simulink model "flightControlSystem"  (R2024b)
settings: Solver=ode3  StartTime=0  StopTime=TFinal  FixedStep=Ts  RelTol=1e-3  EnableMultiTasking=on
undefined symbols (not defined in the file): codertarget, completed, Controller, controller_selector, DiscIntNeverNeededParam, Discrete, distance, Estimator, filter_coef, g, gray, init, orient_ref, pos_ref, Sensors, Time, time_outside_line, Ts, var_acc_angle_N, var_bias_gyr_N, var_gyro_p_N, Vehicle, y
libraries: simulink x42, matrix_library x5, slpidlib x4, ctrlSharedLib x4, sharedtransform x3, parrotlib x1, visiongeotforms x1, simulink_extras x1
(part 3 of 3)

== system flightControlSystem/Control System/State Estimator/XY Position Estimator/EstimatorVelocity/AccelerationHandling ==
  dxy_estimin : Inport
  sensorIMU_datin : Inport  Port=2
  orient_estimin : Inport  Port=3
  Z_estimin : Inport  Port=4
  Add : Sum  Inputs=-+
  Bus Selector1 : BusSelector  OutputSignals=ddx,ddy,ddz
  Deactivate Acceleration If OF is not used due to low altitude : simulink/Logic and Bit Operations/Compare To Constant  relop=<=  const=Estimator.pos.opticalFlowZMax  OutDataTypeStr=boolean
  Logical Operator : Logic  Operator=OR  AllPortsSameDT=off  OutDataTypeStr=boolean
  Mux6 : Mux  Inputs=3
  Product : Product  Inputs=3
  Product1 : Product  Multiplication=Matrix(*)
  Rotation Angles to Direction Cosine Matrix : sharedtransform/Rotation Angles to Direction Cosine Matrix  rotationOrder=ZYX  aMode=aMode
  SelectPlanarddxy : Selector  InputPortWidth=3  IndexOptions=Index vector (dialog)  Indices=[1 2]  OutputSizes=1
  Selector : Selector  InputPortWidth=2  IndexOptions=Index vector (dialog)  Indices=1  OutputSizes=1
  Selector1 : Selector  InputPortWidth=2  IndexOptions=Index vector (dialog)  Indices=2  OutputSizes=1
  do not use acc if optical flow never available (Note OF@60Hz but ZOH to 200!) : simulink/Logic and Bit Operations/Compare To Constant  relop=~=  const=0  OutDataTypeStr=boolean
  do not use acc if optical flow never available (Note OF@60Hz but ZOH to 200!)1 : simulink/Logic and Bit Operations/Compare To Constant  relop=~=  const=0  OutDataTypeStr=boolean
  gainaccinput1 : Gain  OutDataTypeStr=single
  gravity : Constant  Value=[0 0 -g]
  acceleration_world : Outport  OutDataTypeStr=single  VectorParamsAs1DForOutWhenUnconnected=off
  wires:
  do not use acc if optical flow never available (Note OF@60Hz but ZOH to 200!)1/1 -> Logical Operator/2
  do not use acc if optical flow never available (Note OF@60Hz but ZOH to 200!)/1 -> Logical Operator/1
  Logical Operator/1 -> Product/1
  Selector1/1 -> do not use acc if optical flow never available (Note OF@60Hz but ZOH to 200!)1/1
  Selector/1 -> do not use acc if optical flow never available (Note OF@60Hz but ZOH to 200!)/1
  dxy_estimin/1 -> Selector1/1, Selector/1
  Product/1 -> acceleration_world/1
  Deactivate Acceleration If OF is not used due to low altitude/1 -> Product/3
  Z_estimin/1 -> Deactivate Acceleration If OF is not used due to low altitude/1
  Add/1 -> SelectPlanarddxy/1
  Product1/1 -> Add/1
  gravity/1 -> Product1/2
  SelectPlanarddxy/1 -> gainaccinput1/1
  Bus Selector1/3 -> Mux6/3  "<ddz>"
  Bus Selector1/1 -> Mux6/1  "<ddx>"
  sensorIMU_datin/1 -> Bus Selector1/1
  Mux6/1 -> Add/2
  Bus Selector1/2 -> Mux6/2  "<ddy>"
  orient_estimin/1 -> Rotation Angles to Direction Cosine Matrix/1
  Rotation Angles to Direction Cosine Matrix/1 -> Product1/1
  gainaccinput1/1 -> Product/2

== system flightControlSystem/Control System/State Estimator/XY Position Estimator/EstimatorVelocity/Angular velocity compensation for optical flow ==
  note: Optical flow readings are affected by both linear and angular velocity of the drone. We need to subtract the effect of angular velocity before using the flow data
  z_estimate : Inport
  Angular velocity w/o bias : Inport  Port=2
  Abs : Abs  SaturateOnIntegerOverflow=off
  Data Type Conversion : DataTypeConversion  SaturateOnIntegerOverflow=off  RndMeth=Floor
  Demux : Demux  Outputs=2
  Gain1 : Gain  Gain=-1
  Mux : Mux  Inputs=2
  Selector : Selector  InputPortWidth=3  IndexOptions=Index vector (dialog)  Indices=[1 2]  OutputSizes=1
  prod : Product  Inputs=**
  angular velocity correction : Outport
  wires:
  Gain1/1 -> Mux/1
  Mux/1 -> Data Type Conversion/1
  Demux/2 -> Gain1/1
  Data Type Conversion/1 -> angular velocity correction/1
  prod/1 -> Demux/1
  z_estimate/1 -> Abs/1
  Demux/1 -> Mux/2
  Selector/1 -> prod/2
  Abs/1 -> prod/1
  Angular velocity w/o bias/1 -> Selector/1

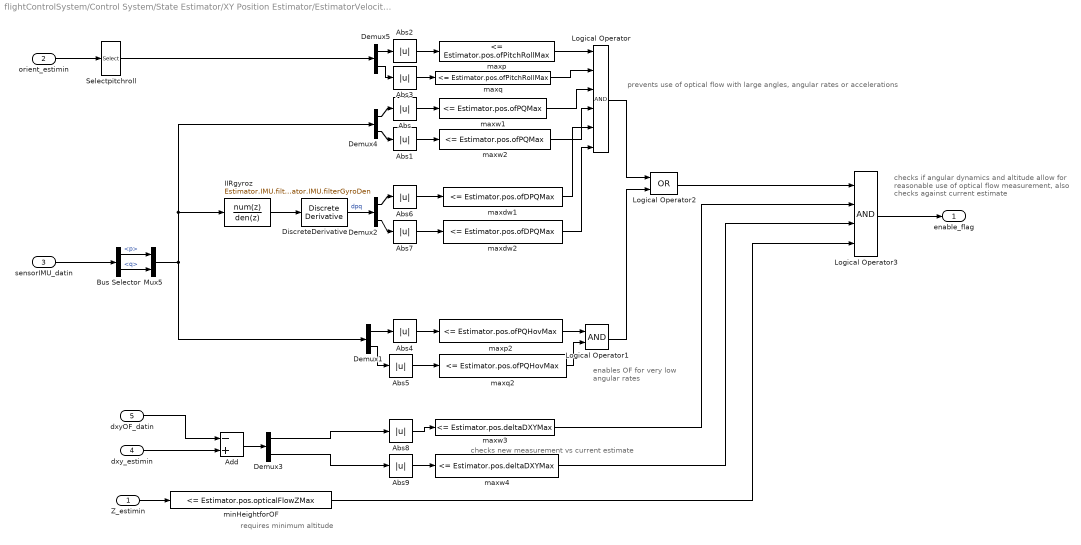
== system flightControlSystem/Control System/State Estimator/XY Position Estimator/EstimatorVelocity/DataHandling ==
  note: prevents use of optical flow with large angles, angular rates or accelerations
  note: enables OF for very
      | low angular rates
  note: checks if angular dynamics and altitude allow for
      | reasonable use of optical flow measurement,
      | also checks against current estimate
  note: checks new measurement vs current estimate
  note: requires minimum altitude
  Z_estimin : Inport
  orient_estimin : Inport  Port=2
  sensorIMU_datin : Inport  Port=3
  dxy_estimin : Inport  Port=4
  dxyOF_datin : Inport  Port=5
  Abs{,1..9} (10 alike) : Abs  SaturateOnIntegerOverflow=off
  Add : Sum  Inputs=-+
  Bus Selector : BusSelector  OutputSignals=p,q
  Demux{1..5} (5 alike) : Demux  Outputs=2
  DiscreteDerivative : simulink/Discrete/Discrete Derivative  gainval=1.0  ICPrevScaledInput=0.0  OutMin=[]  OutMax=[]  OutDataType=fixdt(1, 16)  OutScaling=2^-10  DoSatur=off
  IIRgyroz : DiscreteFilter  Numerator=Estimator.IMU.filterGyroNum  Denominator=Estimator.IMU.filterGyroDen
  Logical Operator : Logic  Inputs=6  AllPortsSameDT=off  OutDataTypeStr=boolean
  Logical Operator1 : Logic  AllPortsSameDT=off  OutDataTypeStr=boolean
  Logical Operator2 : Logic  Operator=OR  AllPortsSameDT=off  OutDataTypeStr=boolean
  Logical Operator3 : Logic  Inputs=4  AllPortsSameDT=off  OutDataTypeStr=boolean
  Mux5 : Mux  Inputs=2
  Selectpitchroll : Selector  InputPortWidth=3  IndexOptions=Index vector (dialog)  Indices=[2 3]  OutputSizes=1
  maxdw1 : simulink/Logic and Bit Operations/Compare To Constant  relop=<=  const=Estimator.pos.ofDPQMax  OutDataTypeStr=boolean
  maxdw2 : simulink/Logic and Bit Operations/Compare To Constant  relop=<=  const=Estimator.pos.ofDPQMax  OutDataTypeStr=boolean
  maxp : simulink/Logic and Bit Operations/Compare To Constant  relop=<=  const=Estimator.pos.ofPitchRollMax  OutDataTypeStr=boolean
  maxp2 : simulink/Logic and Bit Operations/Compare To Constant  relop=<=  const=Estimator.pos.ofPQHovMax  OutDataTypeStr=boolean
  maxq : simulink/Logic and Bit Operations/Compare To Constant  relop=<=  const=Estimator.pos.ofPitchRollMax  OutDataTypeStr=boolean
  maxq2 : simulink/Logic and Bit Operations/Compare To Constant  relop=<=  const=Estimator.pos.ofPQHovMax  OutDataTypeStr=boolean
  maxw1 : simulink/Logic and Bit Operations/Compare To Constant  relop=<=  const=Estimator.pos.ofPQMax  OutDataTypeStr=boolean
  maxw2 : simulink/Logic and Bit Operations/Compare To Constant  relop=<=  const=Estimator.pos.ofPQMax  OutDataTypeStr=boolean
  maxw3 : simulink/Logic and Bit Operations/Compare To Constant  relop=<=  const=Estimator.pos.deltaDXYMax  OutDataTypeStr=boolean
  maxw4 : simulink/Logic and Bit Operations/Compare To Constant  relop=<=  const=Estimator.pos.deltaDXYMax  OutDataTypeStr=boolean
  minHeightforOF : simulink/Logic and Bit Operations/Compare To Constant  relop=<=  const=Estimator.pos.opticalFlowZMax  OutDataTypeStr=boolean
  enable_flag : Outport  VectorParamsAs1DForOutWhenUnconnected=off
  wires:
  minHeightforOF/1 -> Logical Operator3/4
  IIRgyroz/1 -> DiscreteDerivative/1
  Mux5/1 -> Demux1/1, Demux4/1, IIRgyroz/1
  maxw4/1 -> Logical Operator3/3
  maxw3/1 -> Logical Operator3/2
  dxyOF_datin/1 -> Add/1
  Demux3/2 -> Abs9/1
  Demux3/1 -> Abs8/1
  dxy_estimin/1 -> Add/2
  Add/1 -> Demux3/1
  Abs9/1 -> maxw4/1
  Abs8/1 -> maxw3/1
  Logical Operator2/1 -> Logical Operator3/1
  Logical Operator3/1 -> enable_flag/1
  DiscreteDerivative/1 -> Demux2/1  "dpq"
  Demux2/2 -> Abs7/1
  Demux2/1 -> Abs6/1
  Abs7/1 -> maxdw2/1
  Abs6/1 -> maxdw1/1
  Logical Operator1/1 -> Logical Operator2/2
  Demux1/2 -> Abs5/1
  Demux1/1 -> Abs4/1
  Abs5/1 -> maxq2/1
  Abs4/1 -> maxp2/1
  Abs3/1 -> maxq/1
  Abs2/1 -> maxp/1
  Demux4/2 -> Abs1/1
  Demux4/1 -> Abs/1
  Abs1/1 -> maxw2/1
  Abs/1 -> maxw1/1
  Z_estimin/1 -> minHeightforOF/1
  Logical Operator/1 -> Logical Operator2/1
  maxw1/1 -> Logical Operator/3
  Bus Selector/1 -> Mux5/1  "<p>"
  Selectpitchroll/1 -> Demux5/1
  sensorIMU_datin/1 -> Bus Selector/1
  maxq2/1 -> Logical Operator1/2
  Bus Selector/2 -> Mux5/2  "<q>"
  maxp/1 -> Logical Operator/1
  maxw2/1 -> Logical Operator/4
  orient_estimin/1 -> Selectpitchroll/1
  maxdw1/1 -> Logical Operator/5
  maxdw2/1 -> Logical Operator/6
  maxq/1 -> Logical Operator/2
  Demux5/1 -> Abs2/1
  Demux5/2 -> Abs3/1
  maxp2/1 -> Logical Operator1/1

== system flightControlSystem/Control System/State Estimator/XY Position Estimator/EstimatorVelocity/xy velocity w//o angular velocity compensation ==
  note: Optical flow raw readings are converted to velocity in m/s based on the estimated altitude
  optical_flow : Inport
  z_estimate : Inport  Port=2
  " " : Product  Inputs=**
  Compare To Constant : simulink/Logic and Bit Operations/Compare To Constant  relop=<  const=200*4  OutDataTypeStr=boolean
  Counter Free-Running : simulink/Sources/Counter Free-Running  NumBits=32  tsamp=-1
  Gain : Gain  Gain=-1
  Select dxy : Selector  InputPortWidth=3  IndexOptions=Index vector (dialog)  Indices=[1 2]  OutputSizes=1
  Switch : Switch  Criteria=u2 > Threshold  SaturateOnIntegerOverflow=off  InputSameDT=off
  opticalFlowErrorCorrect : Gain  Gain=1.15
  optical_flow_dx_dy : Outport
  wires:
  Select dxy/1 -> optical_flow_dx_dy/1  "optical_flow_dx_dy"
  " "/1 -> opticalFlowErrorCorrect/1
  opticalFlowErrorCorrect/1 -> Switch/3
  Gain/1 -> " "/2
  Switch/1 -> Select dxy/1
  Counter Free-Running/1 -> Compare To Constant/1
  Compare To Constant/1 -> Switch/2
  optical_flow/1 -> " "/1, Switch/1
  z_estimate/1 -> Gain/1

== matlab function flightControlSystem/Image Processing System/soluzione3/fitness Function ==
  data: time_outside_line_in input; time_outside_line output; u input; circleDetected input; total_time input; completed output; distance output
function [time_outside_line,completed,distance] = fcn(time_outside_line_in, u, circleDetected, total_time)

pixels=sum(sum(u(59:61,79:81)));
completed=double(circleDetected);

%counter for the tile outside the line
if(pixels<=4 && circleDetected==0 && total_time>20)
    time_outside_line=time_outside_line_in+1;
else
    time_outside_line=time_outside_line_in;
end

%distance in pixels from the line using circles with center in (100, 100)
%and radius r
distance=0;
if (u(60,80)==0 && total_time>20 && circleDetected==0)
    radius=1;   
    while distance==0
        for t=0:7
            if u(60+round((radius*cos(t*(pi/4)))),80+round((radius*sin(t*(pi/4)))))==1
            distance=radius;
            end
        end
        radius=radius+1;
        if(radius==60)
            distance=radius;
        end
    end
end

== matlab function flightControlSystem/Control System/Controller/Position Controller/Position error transformation (Earth to Body frame) ==
  data: yaw input; xy_err_earth input; xy_err_body output
function xy_err_body = fcn(yaw,xy_err_earth)

transformation = [cos(yaw), sin(yaw); -sin(yaw),  cos(yaw)];
xy_err_body = transformation * xy_err_earth;


end

== matlab function flightControlSystem/Image Processing System/soluzione3/lineFollower ==
  data: next_direction_in input; circle_detected input; u input; next_direction output; t input; mode_in input; theta output; u_out output; x output; mode output
function [next_direction,theta, u_out,x, mode]= fcn(next_direction_in, circle_detected, u, t, mode_in)
    mode=mode_in;
    x=0;
    next_direction=next_direction_in;
    u(80:end,1:end)=0; %% black out the part behind the drone
    %%front
    front= sum(sum(u(21:52,70:90))); %11:52
    front_left = sum(sum(u(11:42,80:90)));
    front_right = sum(sum(u(11:42,70:80)));
    center= sum(sum(u(52:80,67:93)));
    center_left=sum(sum(u(60,74:80))); % rows 52:60  cols 74-80
    center_right =sum(sum(u(60,80:86)));% rows 52:60 cols 80-86
    left =sum(sum(u(31:41,45:55)));
    right = sum(sum(u(31:41,105:115)));
    if(t<=10) %take-off
        theta=0;
        next_direction=0;
        u_out=u;
   
    else
        u_out=u;
        theta=0;
        % front rectangle
        u_out(11:52,70)=ones(42,1);
        u_out(11:52,90)=ones(42,1);
        u_out(11,70:90)=ones(1,21);
        u_out(52,70:90)=ones(1,21);

        % center rectangle
        u_out(52:80,67)=ones(29,1);%move
        u_out(52:80,93)=ones(29,1);% move
        u_out(52,67:93)=ones(1,27);%move
        u_out(80,67:93)=ones(1,27);%move

        % sides
        % left
        u_out(41,45:55)=1;
        u_out(31,45:55)=1;
        u_out(31:41,45)=ones(11,1);
        u_out(31:41,55)=ones(11,1);
        u_out(42:85,65)=1;
        % right
        u_out(41,105:115)=1;
        u_out(31,105:115)=1;
        u_out(31:41,115)=ones(11,1);
        u_out(31:41,105)=ones(11,1);
        u_out(42:85,95)=1;
   
        if mode == 0 % take-off
            if(u(60,80) == 1)
                if is_on_the_line(center,18) == 1 && is_on_the_line(front,42) == 1
                    mode=1;
                elseif(sum(sum(u(20:100,1:80))) < sum(sum(u(20:100,81:160))))
                    next_direction = 1;
                    mode = 2;
                else
                    next_direction = -1;
                    mode = 2;
                end
            end
        end

        if circle_detected == 1
            mode = 5;
        end
        
        if mode == 1 %on the line
            theta = 0;

            if(left>0)
                next_direction=-1;
            elseif(right>0)
                next_direction=1;
            end

            %angle micro adjustments
            if front_left> front_right
                theta = 0.01*(front_left-front_right)*(pi/180);
            elseif front_right> front_left
                theta = -0.01*(front_right-front_left)*(pi/180);
            end

            %position micro adjustment
            if(center_right==center_left)
                x=0;
            elseif(center_right>center_left)
                x=-1;
            elseif(center_right<center_left)
                x=1;
            end
            left_line = sum(sum(u(42:65,60)));
            right_line = sum(sum(u(42:65,100)));
            top_matrix = sum(sum(u(11:21,79:81)));
            if(u(42,76) == 0 || u(42,84) == 0) && next_direction ~= 0 && ...
                    (top_matrix == 0 || (top_matrix > 0 && (u(11,55) + u(11,105) > 0 || left_line + right_line > 0)))
                next_direction=confirm_direction(sum(sum(u(42:85,60))),sum(sum(u(42:85,100))),next_direction);
                mode=2;
            end
        elseif  mode == 2
            theta = next_direction*(pi/180);

            if(is_on_the_line(front,31)==1 )%|| u(30,80)==1) % fix fail SA_2
                next_direction=0;
                mode=1;
            end
        end

    end
end



function y= is_on_the_line(n,h)
    if n <= h*20 && n >= h*18
        y = 1;
    else
        y=0;
    end
end

function direction= confirm_direction(left, right,dir)
direction=dir;
if(left>0 && right == 0)
    direction=-1;
elseif(right>0 && left == 0)
    direction=1;
end

end


%  if(u(42,76) == 0 || u(42,84) == 0) && next_direction ~= 0 && ...
       %      (sum(sum(u(11:21,79:81))) == 0 || (sum(sum(u(11:21,79:81))) > 0 && u(11,55) + u(11,105) > 0) || (sum(sum(u(11:21,79:81))) && sum(sum(u(42:65,60))) + sum(sum(u(42:65,100))) > 0))
       %      next_direction=confirm_direction(sum(sum(u(42:85,60))),sum(sum(u(42:85,100))),next_direction);% test to confirm direction
       %      mode=2;
       %      %[next_direction,mode]= overwrite(u,next_direction,mode);
       % end


% function [direction, mode]= overwrite(u,direction_in,mode_in)
% line = sum(u(63,68:90));
% left_point= u(60,68);
% right_point= u(60,92);
% bottom_left_point= u(70,68);
% bottom_right_point= u(70,92);
% direction = direction_in;
% mode = mode_in;
% if(line+left_point+right_point+bottom_left_point+bottom_right_point==0)
%     direction=0;
%     mode=1;
% end
% 
% end

== matlab function flightControlSystem/Image Processing System/soluzione3/speedAndDirection ==
  data: circleDetect_in input; speed input; y output; theta input; x input; mode input; t input
function y  = fcn( circleDetect_in, speed, theta, x, mode, t)
p=1/3;
if(t<10)
    circleDetected=0;
     y = [0,0,0,circleDetected];
else
    circleDetected=circleDetect_in;
    
if mode==1   
    s=0.7;
    if(speed<0)
        s=0.1;
    end
    
elseif mode==2
    s=0;
    x=0;
else
    s=0;
end

    y=[s,x,theta,circleDetected]; 


end

== matlab function flightControlSystem/Control System/Path Planning/soluzione3/MATLAB Function ==
  data: theta output; u input; y output; x output; circleDetected output
function [theta,y, x, circleDetected]= fcn( u)
y=u(1);
x=u(2);

theta= u(3);
circleDetected = u (4);
%x = 0;%*sin(theta);
%y = speed;%*cos(theta);
%x=data*cos(theta/180*pi);
%y=data*sin(theta/180*pi);

== stateflow chart flightControlSystem/Control System/Path Planning/soluzione3/Chart ==
  state hover
    x_out=y*sin(thetaValue)-x*(cos(thetaValue));
    y_out=y*cos(thetaValue)+x*(sin(thetaValue));
  state landing
    x_out=0;
    y_out=0;
    z=0;
  (default) -> hover
  hover -> landing : [circleDetected==1]
  data: thetaValue input; y input; x input; circleDetected input; y_out output; x_out output; z output

== matlab function flightControlSystem/Control System/Path Planning/Soluzione1/MATLAB Function ==
  data: u input; y output; x output; circleDetected output
function [y, x, circleDetected]= fcn(u)

x=u(2);
y = u(1);
circleDetected= u(3);

== matlab function flightControlSystem/Image Processing System/soluzione3/detectCircle1 ==
  data: u input; y output
function y = fcn(u)

y=0;
i=0;
columns_counter=0;
rows_counter=0;
u=imbinarize(u);
w=u;
u=u(21:100,61:100); % cols 41:120 rows 21:100
for r= 1:80
    for c= 1:40
        if u(r,c)==1
            i=i+1;
            columns_counter=columns_counter+c;
            rows_counter=rows_counter+r;
        end
    end
end
if i==0
    y=0;
    return
end
center_column=(columns_counter/i)+60;
center_row=(rows_counter/i)+20;
rho=15;
for theta= 0:62
    if w(round((rho*cos(theta/10)+center_row)), round((rho*sin(theta/10)+center_column)))==0
        y=0;
        return
    end
end
for theta= 0:62
    if w(round(((rho+6)*cos(theta/10)+center_row)), round(((rho+6)*sin(theta/10)+center_column)))==1 
        y=0;
        return
    end
end
    y=1;
end

== stateflow chart flightControlSystem/Control System/Path Planning/Soluzione1/Chart ==
  state hover
    x_out=x;
    y_out=y;
  state landing
    x_out=0;
    y_out=0;
    z=5;
  (default) -> hover
  hover -> landing : [circleDetected==1]
  data: data input; y input; x input; circleDetected input; y_out output; x_out output; z output

== matlab function flightControlSystem/Image Processing System/Soluzione1/detect circle ==
  data: u input; y output
function y = fcn(u)
y=0;
i=0;
columns_counter=0;
rows_counter=0;
u=imbinarize(u);
w=u;
u=u(21:100,41:120);
for r= 1:80
    for c= 1:80
        if u(r,c)==1
            i=i+1;
            columns_counter=columns_counter+c;
            rows_counter=rows_counter+r;
        end
    end
end
if i==0
    y=0;
    return
end
center_column=(columns_counter/i)+40;
center_row=(rows_counter/i)+20;
rho=15;
for theta= 0:62
    if w(round((rho*cos(theta/10)+center_row)), round((rho*sin(theta/10)+center_column)))==0
        y=0;
        return
    end
end
    y=1;
end

== matlab function flightControlSystem/Image Processing System/Soluzione1/MATLAB Function ==
  data: control_matrix_in input; control_matrix_out output; binaryImage input; last_direction input; x_in input; y_in input; filteredBinaryImage output boolean; x_out output; y_out output
function [control_matrix_out, filteredBinaryImage,x_out, y_out] = fcn( control_matrix_in, binaryImage, last_direction, x_in, y_in)

 binaryImage=imbinarize(binaryImage);

if(last_direction(1)==1)
    y_in=y_in-1;
    control_matrix_in(y_in-5:y_in+60,x_in-20:x_in+20)=ones(66,41);

elseif(last_direction(1)==-1)
    y_in=y_in+1;
    control_matrix_in(y_in-55:y_in-5,x_in-20:x_in+20)=ones(51,41);

elseif(last_direction(2)==-1)
    x_in=x_in-1;
    control_matrix_in(y_in-15:y_in+25,x_in:x_in+80)=ones(41,81);
    
elseif(last_direction(2)==1)
    x_in=x_in+1;
    control_matrix_in(y_in-15:y_in+25,x_in-80:x_in)=ones(41,81);
   
end
control_matrix_out=control_matrix_in;
x_out=x_in;
y_out=y_in;
filteredBinaryImage = filterImage(control_matrix_in,x_in-80,y_in-60,binaryImage);
end

function filterImage=filterImage(control_matrix,x,y,im)
    for r=0:119
        for c=0:159
            if(control_matrix(y+r,x+c)==1)
                im(r+1,c+1)=0;
            end
        end
    end
    filterImage=im;
end

== matlab function flightControlSystem/Image Processing System/Soluzione1/direction ==
  data: circle input; y output size=[1 2]; init_directions input; bottom input; top input; left input; right input; t input; last_direction_in input; circleDetected output; last_direction_out output
function [y,circleDetected, last_direction_out] = fcn(circle, init_directions, bottom, top, left, right, t, last_direction_in)
% last_direction: 1=up
% 2 = down
% 3 = left
% 4= right

 last_direction_out=last_direction_in;
 up_down = init_directions(1);
 left_right=init_directions(2);
 
if(t<10)
    y=[0,0];
    circleDetected=0;
else
    circleDetected=circle;    
   
    if (last_direction_in==1)
        [up_down, left_right,last_direction_out] = check_up(bottom, top, left, right, last_direction_in);
    elseif (last_direction_in==2)
        [up_down, left_right,last_direction_out] = check_bottom(bottom, top, left, right, last_direction_in);
    elseif (last_direction_in==3)
        [up_down, left_right,last_direction_out] = check_left(bottom, top, left, right, last_direction_in);
    elseif (last_direction_in==4)
        [up_down, left_right,last_direction_out] = check_right(bottom, top, left, right, last_direction_in);
    
    end

    y=[up_down,left_right];

end
end

function [up_down, left_right,last_direction_out] = check_up(bottom, top, left, right, last_direction_in)
    if (top>=150)%=bottom && top>0)
        up_down=1;
        left_right = 0;
        last_direction_out=1;
    elseif (right>=left && right>0)
        left_right=1;
        up_down = 0;
        last_direction_out=4;
    elseif (left>=right && left>0)
        left_right=-1;
        up_down = 0;
        last_direction_out=3;
    else
        left_right=0;
        up_down = 0;
        last_direction_out=last_direction_in;
     end
 end

function [up_down, left_right,last_direction_out] = check_bottom(bottom, top, left, right, last_direction_in)
    if (bottom>=150)%=top && bottom>0)
       up_down=-1;
       left_right = 0;
       last_direction_out=2;
    elseif (right>=left && right>0)
        left_right=1;
        up_down = 0;
        last_direction_out=4;
    elseif (left>=right && left>0)
        left_right=-1;
        up_down = 0;
        last_direction_out=3;
    else
        left_right=0;
        up_down = 0;
        last_direction_out=last_direction_in;
    end
end

function [up_down, left_right,last_direction_out] = check_left(bottom, top, left, right, last_direction_in)
    if (left>=200)%=right && left>0)
        up_down=0;
        left_right = -1;
        last_direction_out=3;
    elseif (bottom>=top && bottom>0)
        up_down=-1;
        left_right = 0;
        last_direction_out=2;
    elseif (top>=bottom && top>0)
         up_down=1;
         left_right = 0;
         last_direction_out=1;
    else
         left_right=0;
         up_down = 0;
         last_direction_out=last_direction_in;
    end
end

function [up_down, left_right,last_direction_out] = check_right(bottom, top, left, right, last_direction_in)
    if (right>=200)%=left && right>0)
        up_down=0;
        left_right = 1;
        last_direction_out=4;
    elseif (bottom>=top && bottom>0)
        up_down=-1;
        left_right = 0;
        last_direction_out=2;
    elseif (top>=bottom && top>0)
        up_down=1;
        left_right = 0;
        last_direction_out=1;
    else
        left_right=0;
        up_down = 0;
        last_direction_out=last_direction_in;
    end
end

== matlab function flightControlSystem/Image Processing System/Soluzione1/MATLAB Function1 ==
  data: matrix_bottom input; bottom output; top output; matrix_top input; matrix_left input; matrix_right input; left output; right output
function [bottom, top, left, right] = fcn(matrix_bottom, matrix_top ,matrix_left,matrix_right)

bottom = sum(sum(matrix_bottom(:,:)));
top = sum(sum(matrix_top(:,:)));
left = sum(sum(matrix_left(:,:)));
right = sum(sum(matrix_right(:,:)));

== matlab function flightControlSystem/Image Processing System/soluzione2/detect circle ==
  data: u input; y output
function y = fcn(u)

y=0;
i=0;
columns_counter=0;
rows_counter=0;
u=imbinarize(u);
w=u;
u=u(21:100,21:115); % cols 41:120 rows 21:100
for r= 1:80
    for c= 1:95
        if u(r,c)==1
            i=i+1;
            columns_counter=columns_counter+c;
            rows_counter=rows_counter+r;
        end
    end
end
if i==0
    y=0;
    return
end
center_column=(columns_counter/i)+20;
center_row=(rows_counter/i)+20;
rho=15;
for theta= 0:62
    if w(round((rho*cos(theta/10)+center_row)), round((rho*sin(theta/10)+center_column)))==0
        y=0;
        return
    end
end
for theta= 0:62
    if w(round(((rho+6)*cos(theta/10)+center_row)), round(((rho+6)*sin(theta/10)+center_column)))==1 
        y=0;
        return
    end
end
    y=1;
end

== matlab function flightControlSystem/Image Processing System/soluzione2/MATLAB Function ==
  data: u input; y output
function y = fcn(u)
u=imbinarize(u);
u(131:200,:)=zeros(70,200);
y = u;

== matlab function flightControlSystem/Image Processing System/soluzione2/MATLAB Function1 ==
  data: whitePixels_in input; last_theta input; theta_in input; u input; whitePixels output; turning_in input; t input; theta output; u_out output; turning output
function [whitePixels,theta, u_out,turning] = fcn(whitePixels_in, last_theta, theta_in, u, turning_in, t)
 turning=turning_in;
if(t<=20)
    theta=theta_in;
    whitePixels=whitePixels_in;
    %u=imbinarize(u);
    u_out=u;
   
    % u_out(51:80,86)=ones(30,1);
    % u_out(51:80,115)=ones(30,1);
    % u_out(51,86:115)=ones(1,30);
    % u_out(80,86:115)=ones(1,30);
    % u_out(51:90,81)=ones(40,1);%move
    % u_out(51:90,120)=ones(40,1);% move
    % u_out(51,81:120)=ones(1,40);%move
    % u_out(86,81:120)=ones(1,40);%move
    %%%%%%%%%%%%%%%%%%%%%%%%

   
    %%%%%%%%%%%%%%%%%%%%%%
else
    %u=imbinarize(u);
    n=3;%step size (degrees)
    u_out=u;
    u_out(44:47,99)=ones(4,1);
    u_out(44:47,102)=ones(4,1);
    u_out(44,99:102)=ones(1,4);
    u_out(47,99:102)=ones(1,4);
    u_out(41:80,86)=ones(40,1);%move
    u_out(41:80,115)=ones(40,1);% move
    u_out(41,86:115)=ones(1,30);%move
    u_out(80,86:115)=ones(1,30);%move

    u_out(1,70:75)=ones(1,6);
    u_out(110,70:75)=ones(1,6);
    u_out(1,125:130)=ones(1,6);
    u_out(110,125:130)=ones(1,6);
    u_out(1:110,75)=ones(110,1);
    u_out(1:110,70)=ones(110,1);
    u_out(1:110,130)=ones(110,1);
    u_out(1:110,125)=ones(110,1);
    %left1
    u_out(1:90,1)=ones(90,1);
    u_out(1:90,80)=ones(90,1);
    u_out(1,1:80)=ones(1,80);
    u_out(90,1:80)=ones(1,80);
    %right1
    u_out(1:90,121)=ones(90,1);
    u_out(1:90,200)=ones(90,1);
    u_out(1,121:200)=ones(1,80);
    u_out(90,121:200)=ones(1,80);

    %w=u(51:80,86:115);
    w=u(44:47,99:102);
    
whitePixels= sum(sum(w(:)));
left2=sum(sum(u(1:110,70:75)));%  1:90
right2=sum(sum(u(1:110,125:130)));

if((whitePixels> whitePixels_in|| whitePixels>=4) || ((left2+right2==0)&&t>=30))
%if(whitePixels >= 150)

    theta=theta_in;
    turning=0;
elseif(left2+right2==0 && t<30)
    theta = theta_in+(n*pi/180);
    turning=1;
else
    if(u(90,100)==1&& whitePixels==0&& t>30 && turning == 0)
        theta=theta_in;
        turning=0;
    else
    left1=sum(sum(u(1:90,1:80)));% 1:80 => 1:70
    %left2=sum(sum(u(1:90,70:75)));
    left = left1+left2;

    right1=sum(sum(u(1:90,121:200)));% 121:200 => 131:200
    %right2=sum(sum(u(1:90,125:130)));
    right=right1+right2;
%%%%%%%%%%%%%
    if theta_in <last_theta && turning==1
        theta = theta_in-(n*pi/180);
    elseif theta_in >last_theta && turning==1
        theta = theta_in+(n*pi/180);
    else
 %%%%%%%%%%%%%
    if( left>= right)
        theta = theta_in-(n*pi/180);
        turning=1;
    else
        theta = theta_in+(n*pi/180);
        turning=1;
    end%%%%%%%%%%%%%
    end
     if(u(100,100)==0 && t>30 && left+right==0 && whitePixels==0)
        theta = theta_in-(n*pi/180);
        turning=1;
     end
    end
   
end
end

== matlab function flightControlSystem/Image Processing System/soluzione2/fitness Function ==
  data: time_outside_line_in input; time_outside_line output; u input; circleDetected input; total_time input; completed output; distance output
function [time_outside_line,completed,distance] = fcn(time_outside_line_in, u, circleDetected, total_time)

pixels=sum(sum(u(97:103,97:103)));
completed=double(circleDetected);

%counter for the tile outside the line
if(pixels<=0 && circleDetected==0 && total_time>20)
    time_outside_line=time_outside_line_in+1;
else
    time_outside_line=time_outside_line_in;
end

%distance in pixels from the line using circles with center in (100, 100)
%and radius r
distance=0;
if (u(100,100)==0 && total_time>20 && circleDetected==0)
    radius=1;   
    while distance==0
        for t=0:7
            if u(100+round((radius*cos(t*(pi/4)))),100+round((radius*sin(t*(pi/4)))))>=1
            distance=radius;
            end
        end
        radius=radius+1;
        if(radius==100 || distance >0)
            distance=radius;
        end
    end
end

== matlab function flightControlSystem/Image Processing System/soluzione2/MATLAB Function2 ==
  data: circleDetect_in input; u input; y output; theta input; t input; circleDetected output
function [y,circleDetected] = fcn( circleDetect_in, u, theta, t)
p=1/300;
if(t<10)
    circleDetected=0;
     y = [0,theta];
else
    circleDetected=circleDetect_in;

u=imbinarize(u);
w=u(41:90,86:115);%89:112 more accuracy slower time
%w=u(61:90,86:115);
%w=u(51:80,86:115);
whitePixels=sum(w(:));
if(whitePixels>=100)
    s=max((whitePixels-100)*p,0.4);
    %s=(whitePixels-100)*p;
    y=[s,theta]; 
else
    y = [0,theta]; 
end
end

== stateflow chart flightControlSystem/Control System/Path Planning/Soluzione2/Chart ==
  state hover
    x_out=speed*sin(theta);
    y_out=speed*cos(theta);
  state landing
    x_out=0;
    y_out=0;
    z=5;
  (default) -> hover
  hover -> landing : [circleDetected==1]
  data: speed input; theta input; circleDetected input; y_out output; x_out output; z output

== matlab function flightControlSystem/Control System/Path Planning/Soluzione2/MATLAB Function ==
  data: u input; s output; theta output; circleDetected output
function [s, theta, circleDetected]= fcn(u)

theta=u(2);
s = u(1);
circleDetected= u(3);

== matlab function flightControlSystem/Image Processing System/Soluzione1/fitness Function ==
  data: time_outside_line_in input; time_outside_line output; u input; circleDetected input; total_time input; completed output; distance output
function [time_outside_line,completed,distance] = fcn(time_outside_line_in, u, circleDetected, total_time)
u=imbinarize(u);
pixels=sum(sum(u(55:65,75:85)));
if(total_time<10)
    
    completed=0;
else
completed=double(circleDetected);
end
%counter for the tile outside the line
if(pixels<=0 && circleDetected==0 && total_time>20)
    time_outside_line=time_outside_line_in+1;
else
    time_outside_line=time_outside_line_in;
end

%distance in pixels from the line using circles with center in (100, 100)
%and radius r
distance=0;
if (pixels==0 && total_time>20 && circleDetected==0)
    radius=5;   
    while distance==0
        for t=0:7
            if u(60+round((radius*cos(t*(pi/4)))),80+round((radius*sin(t*(pi/4)))))==1
            distance=radius-4;
            break
            end
        end
        radius=radius+1;
        if(radius==60)
            distance=radius;
        end
    end
end

== stateflow chart flightControlSystem/Image Processing System/soluzione3/Chart ==
  state hover
    %defining the control matrices
    img = img_in;
    img(80:end,1:end)=0;
    front = sum(sum(img(21:52,70:90)));
    front_left = sum(sum(img(11:42,80:90)));
    front_right = sum(sum(img(11:42,70:80)));
    center = sum(sum(img(52:80,67:93)));
    center_left = sum(sum(img(60,74:80)));
    center_right = sum(sum(img(60,80:86)));
    left = sum(sum(img(31:41,45:55)));
    right = sum(sum(img(31:41,105:115)));
    left_half = sum(sum(img(20:100,1:80)));
    right_half = sum(sum(img(20:100,81:160)));
    state on_the_line
      entry:
      next_direction = 0;
      theta = 0;
      during:
      mode = 1;
      theta = angle_adjustment;
      x = position_adjustment;
      next_direction = check_direction;
      exit:
      next_direction = confirm_direction(sum(sum(img(42:85,60))),sum(sum(img(42:85,100))),next_direction);
    state take_off
      mode = 0;
    state turning
      mode = 2;
      theta = next_direction*(pi/180);
    state pick_direction [function]
      (default) -> (junction 66)
      (junction 66) -> (junction 67) [order 1] : [left_half < right_half]
      (junction 66) -> (junction 68) [order 2] : {next_direction = -1;}
      (junction 67) -> (junction 69) : {next_direction = 1;}
      (junction 69) -> (junction 68)
      (junction 68) -> (junction 70)
    (default) -> take_off
    take_off -> on_the_line [order 1] : [t>10 && is_on_the_line(center, 18)==1 && is_on_the_line(front, 42)==1]
    on_the_line -> turning : [check_condition(next_direction)]
    turning -> on_the_line : [is_on_the_line(front,31)==1]
    take_off -> turning [order 2] : [t>10 && ( is_on_the_line(center, 18)==0 || is_on_the_line(front, 42)==0)] {pick_direction}
  state landing
    mode = 5;
    x = 0;
    theta = 0;
  (default) -> hover
  hover -> landing : [circle_detected==1]
  data: n function_input; h function_input; y function_output; left function_input; right function_input; dir function_input; direction function_output; dir function_output; cond function_output; next_direction function_input; ang function_output; pos function_output; circle_detected input; img_in input; next_direction output; theta output; x output; mode output; t input; center local; center_left local; center_right local; front local; front_left local; front_right local; left local; right local; left_half local; right_half local; img local
  function y= is_on_the_line(n,h):
    | function y= is_on_the_line(n,h)
    |     if n <= h*20 && n >= h*18
    |         y = 1;
    |     else
    |         y=0;
    |     end
    | end
  function direction= confirm_direction(left, right,dir):
    | function direction= confirm_direction(left, right,dir)
    |     direction=dir;
    |     if(left>0 && right == 0)
    |         direction=-1;
    |     elseif(right>0 && left == 0)
    |         direction=1;
    |     end
    | end
  function dir= check_direction:
    | function dir= check_direction
    |     if(left > 0)
    |         dir = -1;
    |     elseif(right > 0)
    |         dir = 1;
    |     else 
    |         dir = next_direction;
    |     end
    | end
  function cond = check_condition(next_direction):
    | function cond = check_condition(next_direction)
    |     left_line = sum(sum(img(42:65,60)));
    |     right_line = sum(sum(img(42:65,100)));
    |     top_matrix = sum(sum(img(11:21,79:81)));
    |     cond = (img(42,76) == 0 || img(42,84) == 0) && next_direction ~= 0 && ...
    |             (top_matrix == 0 || (top_matrix > 0 && (img(11,55) + img(11,105) > 0 || left_line + right_line > 0)));
    |       
    | end
  function ang = angle_adjustment:
    | %angle micro adjustments
    | function ang = angle_adjustment
    |     if front_left> front_right
    |         ang = 0.01*(front_left-front_right)*(pi/180);
    |     elseif front_right> front_left
    |         ang = -0.01*(front_right-front_left)*(pi/180);
    |     else
    |         ang = 0;
    |     end
    | end
  function pos = position_adjustment:
    | %position micro adjustment
    | function pos = position_adjustment
    |     if(center_right==center_left)
    |         pos=0;
    |     elseif(center_right>center_left)
    |         pos=-1;
    |     elseif(center_right<center_left)
    |         pos=1;
    |     else
    |         pos = 0;
    |     end
    | end

== matlab function flightControlSystem/Control System/Path Planning/MATLAB Function ==
  data: x input; p output; y input; init parameter
function p = fcn(x, y, init)
    p = [x+init.posNED(1),y+init.posNED(2)];

== stateflow chart flightControlSystem/Image Processing System/soluzione3/Chart1 ==
  state hover
    state on_the_linee
      entry:
      next_direction = 0;
      theta = 0;
      during:
      mode = 1;
      ...
      exit:
      ...
    state take_off
      mode = 0;
    state turning
      mode = 2;
      theta = next_direction*(pi/180);
    (default) -> take_off
    take_off -> on_the_linee [order 1] : [t>10 && is_on_the_line(center, 18)==1 ...
        | && is_on_the_line(front, 42)==1]
    turning -> on_the_linee : [is_on_the_line(front,31)==1]
    on_the_linee -> turning : [check_condition(next_direction)]
    take_off -> turning [order 2] : [t>10 && ( is_on_the_line(center, 18)==0 ...
        |  || is_on_the_line(front, 42)==0)] ...
        | {pick_direction}
  state landing
    mode = 5;
    x = 0;
    theta = 0;
  (default) -> hover
  hover -> landing : [circle_detected==1]
  data: circle_detected input; next_direction output; theta output; x output; mode output; t input; center local; center_left local; center_right local; front local; front_left local; front_right local; left local; right local; left_half local; right_half local; img local

== matlab function flightControlSystem/Image Processing System/MATLAB Function ==
  data: u input; y output
function y = fcn(u)
    y = u;
    y(42:80,57) = 255;   
    y(42:80,103) = 255;
end
